simulink model "power_measurement"  (Simulink 10.0)
settings: Solver=ode45  StartTime=0.0  StopTime=10.0  RelTol=1e-3  EnableMultiTasking=on
libraries: powerlib_extras x1, powerlib x1
settings Model: Creator=samsung  LastModifiedBy=bhisma
settings DataIOCC: LimitDataPoints=on  SignalLoggingSaveFormat=ModelDataLogs
settings OptimizationCC: ExpressionDepthLimit=2147483647
settings DebuggingCC: SolverPrmCheckMsg=warning  FcnCallInpInsideContextMsg=warning  StateNameClashWarn=warning
settings ConfigComp: CovExternalEMLEnable=off

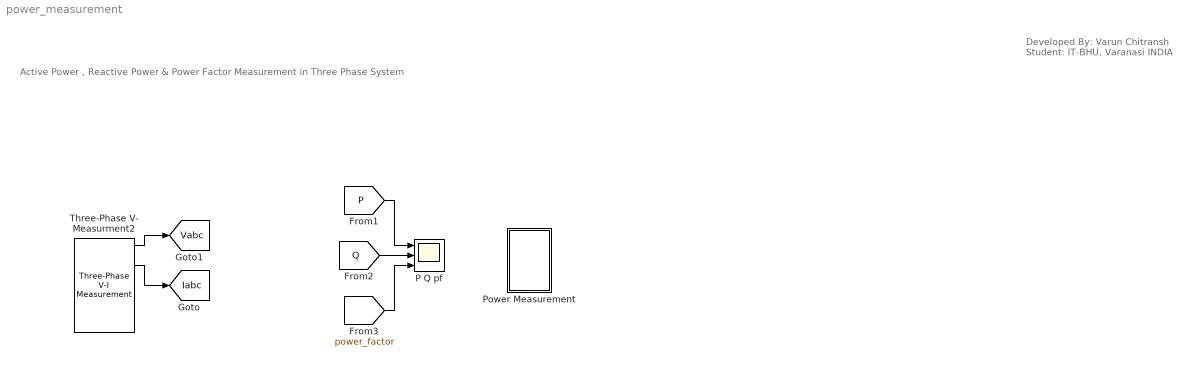
== system power_measurement ==
  note: Developed By: Varun Chitransh
      | Student: IT-BHU, Varanasi INDIA
  note: Active Power , Reactive Power & Power Factor Measurement in Three Phase System
  " Power Measurement" : Subsystem
  P Q pf : Scope  NumInputPorts=3
  Three-Phase V- Measurment2 : powerlib/Measurements/Three-Phase V-I Measurement  SystemSampleTime=-1  VoltageMeasurement=phase-to-ground  SetLabelV=off  LabelV=Vabc  Vpu=off  CurrentMeasurement=yes  SetLabelI=off  LabelI=Iabc  Ipu=off  Pbase=100e6  Vbase=500e3  OutputType=Complex  PhasorSimulation=off  PSBequivalent=0
      settings: SourceProductName=Simscape Electrical
  tag scope: Iabc=global, Vabc=global
  wires:
  [P] -> P Q pf/1
  [Q] -> P Q pf/2
  [power_factor] -> P Q pf/3
  Three-Phase V- Measurment2/1 -> [Vabc]
  Three-Phase V- Measurment2/2 -> [Iabc]

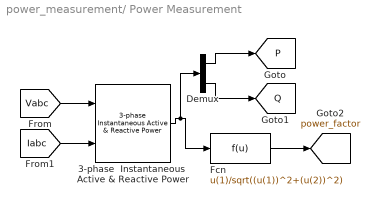
== system power_measurement/ Power Measurement ==
  3-phase  Instantaneous  Active & Reactive Power : powerlib_extras/Measurements/3-phase  Instantaneous  Active & Reactive Power  SystemSampleTime=-1
      settings: SourceProductName=Simscape Electrical  SourceProductBaseCode=PS
  Demux : Demux  Outputs=2
  Fcn : Fcn  Expr=u(1)/sqrt((u(1))^2+(u(2))^2)
  tag scope: P=global, Q=global, power_factor=global
  wires:
  Fcn/1 -> [power_factor]
  Demux/2 -> [Q]
  Demux/1 -> [P]
  3-phase  Instantaneous  Active & Reactive Power/1 -> Demux/1, Fcn/1
  [Iabc] -> 3-phase  Instantaneous  Active & Reactive Power/2
  [Vabc] -> 3-phase  Instantaneous  Active & Reactive Power/1
